simulink model "tp401796"  (Simulink 3.0)
settings: Solver=ode1  SolverMode=SingleTasking  StartTime=0.0  StopTime=t_sim  FixedStep=Ts  RelTol=1e-3
values from neighbouring files (symbols this model uses):
  Ts = 1    [init_PI1_windupless.m]    (also in init_PID1_windupless_tune3.m = 0.5; init_step_resp2.m = 0.2; prev45_0.mat = 0.2; prev45_1.mat = 0.2)
  Umax = 5    [init_PI1_windupless.m]    (also in init_PID1_windupless_tune3.m; init_step_resp2.m; prev45_0.mat; prev45_1.mat)
  Umin = 0    [init_PI1_windupless.m]    (also in init_PID1_windupless_tune3.m; init_step_resp2.m; prev45_0.mat; prev45_1.mat)
libraries: udaq28LT_lib x1
settings Model: LastModifiedBy=mato  ExtModeMexFile=rtwinext  ExtModeTrigDuration=100000  SaveFormat=Matrix  RTWSystemTargetFile=rtwin.tlc  RTWTemplateMakefile=rtwintmf  RTWOptions="-aCCOptimize=1 -aEnforceIntegerDowncast=1 -aExtMode=1 -aFoldNonRolledExpr=1 -aForceParamTrailComments=0 -aGenerateComments=1 -aGenerateReport=0 -aIncDataTypeInIds=0 -aIncHierarchyInIds=0 -aInlineInvariantSignals=0 -aInlinedPrmAccess=\"Literals\" -aLocalBlockOutputs=1 -aMaxRTWIdLen=31 -aPrefixModelToSubsysFcnNames=1 -aRTWVerbose=1 -aRebuildAll=1 -aRollThreshold=5 -aShowEliminatedStatements=1"

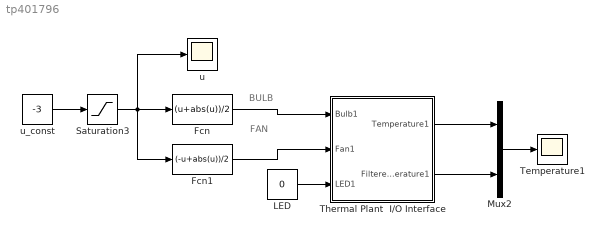
== system tp401796 ==
  note: BULB
  note: FAN
  Fcn : Fcn  Expr=(u+abs(u))/2
  Fcn1 : Fcn  Expr=(-u+abs(u))/2
  LED : Constant  Value=0
  Mux2 : Mux  Inputs=2
  Saturation3 : Saturate  UpperLimit=Umax  LowerLimit=Umin
  Temperature1 : Scope
      settings: TickLabels=on  TimeRange=30  YMin=15  YMax=50  SaveName=yt  DataFormat=Matrix
  Thermal Plant  I/O Interface : Subsystem
      mask Display: disp('Thermo-optical\nPlant\nI/O Interface')
  u : Scope
      settings: TimeRange=180  YMin=-3  YMax=3  SaveName=u  DataFormat=Matrix  Decimation=10  SampleInput=on  SampleTime=Ts
  u_const : Constant  Value=-3
  wires:
  Saturation3/1 -> u/1, Fcn/1, Fcn1/1
  u_const/1 -> Saturation3/1
  Mux2/1 -> Temperature1/1
  Thermal Plant  I/O Interface/1(Temperature1) -> Mux2/1
  Thermal Plant  I/O Interface/2(Filtered  temperature1) -> Mux2/2
  Fcn/1 -> Thermal Plant  I/O Interface/1(Bulb1)
  Fcn1/1 -> Thermal Plant  I/O Interface/2(Fan1)
  LED/1 -> Thermal Plant  I/O Interface/3(LED1)

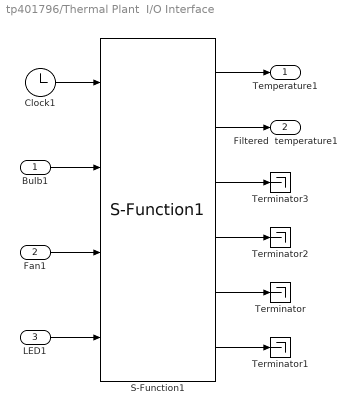
== system tp401796/Thermal Plant  I/O Interface ==
  Bulb1 : Inport  Port=1  PortWidth=-1  SampleTime=-1  DataType=auto
      settings: SignalType=auto
  Fan1 : Inport  Port=2  PortWidth=-1  SampleTime=-1  DataType=auto
      settings: SignalType=auto
  LED1 : Inport  Port=3  PortWidth=-1  SampleTime=-1  DataType=auto
      settings: SignalType=auto
  Clock1 : Clock
      settings: DisplayTime=off  Decimation=10
  S-Function1 : udaq28LT_lib/S-Function1  Priority=1  com_port=COM3  Ts=Ts  events_ot=2  rd_timeout=Ts/2*1000  matlab_prior=ABOVE_NORMAL_PRIORITY  warning=on  printout=off
  Terminator{,1..3} (4 alike) : Terminator
  Temperature1 : Outport  Port=1
  Filtered  temperature1 : Outport  Port=2
  wires:
  S-Function1/1 -> Temperature1/1
  S-Function1/2 -> Filtered  temperature1/1
  Clock1/1 -> S-Function1/1
  Bulb1/1 -> S-Function1/2
  Fan1/1 -> S-Function1/3
  S-Function1/3 -> Terminator3/1
  S-Function1/4 -> Terminator2/1
  S-Function1/5 -> Terminator/1
  S-Function1/6 -> Terminator1/1
  LED1/1 -> S-Function1/4
